simulink model "test_simulation_3_movement"  (R2022a)
settings: Solver=VariableStepAuto  StartTime=0.0  StopTime=1  RelTol=1e-3
libraries: simulink x24, spsMosfetLib x24, spsControlledVoltageSourceLib x4, slpidlib x4, spsPermanentMagnetSynchronousMachineLib x4, spspowerguiLib x1
(part 2 of 2)

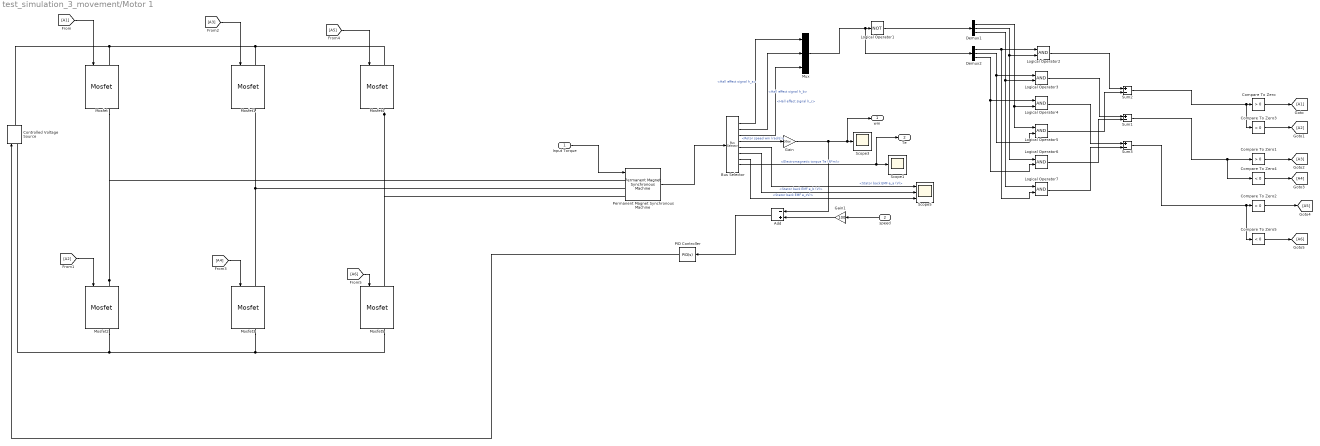
== system test_simulation_3_movement/Motor 1 ==
  Input Torque : Inport
  speed : Inport  Port=2
  Add : Sum  Inputs=-+
  Bus Selector : BusSelector  OutputSignals=Hall effect signal h_a,Hall effect signal h_b,Hall effect signal h_c,Rotor speed wm (rad/s),Stator back EMF e_a (V),Stator back EMF e_b (V),Stator back EMF e_cV),Electromagnetic torque Te (N*m)
  Compare To Zero : simulink/Logic and Bit Operations/Compare To Zero  relop=>  OutDataTypeStr=boolean
  Compare To Zero1 : simulink/Logic and Bit Operations/Compare To Zero  relop=>  OutDataTypeStr=boolean
  Compare To Zero2 : simulink/Logic and Bit Operations/Compare To Zero  relop=>  OutDataTypeStr=boolean
  Compare To Zero3 : simulink/Logic and Bit Operations/Compare To Zero  relop=<  OutDataTypeStr=boolean
  Compare To Zero4 : simulink/Logic and Bit Operations/Compare To Zero  relop=<  OutDataTypeStr=boolean
  Compare To Zero5 : simulink/Logic and Bit Operations/Compare To Zero  relop=<  OutDataTypeStr=boolean
  Controlled Voltage Source : spsControlledVoltageSourceLib/Controlled Voltage Source  Initialize=on  Source_Type=DC  Amplitude=160  Phase=0  Frequency=0  Measurements=None
  Demux1 : Demux  Outputs=3
  Demux2 : Demux  Outputs=3
  Gain : Gain  Gain=30/pi
  Gain1 : Gain  Gain=100
  Logical Operator1 : Logic  Operator=NOT  AllPortsSameDT=off  OutDataTypeStr=boolean
  Logical Operator{2..7} (6 alike) : Logic  AllPortsSameDT=off  OutDataTypeStr=boolean
  Mosfet{,1..5} (6 alike) : spsMosfetLib/Mosfet  Ron=0.1  Lon=0  Rd=0.01  Vfd=0  IC=0  Rs=1e5  Cs=inf  Measurements=on
  Mux : Mux  Inputs=3
  PID Controller : slpidlib/PID Controller  Controller=PID  Form=Parallel  TimeDomain=Continuous-time  UseExternalTs=off  SampleTime=-1  IntegratorMethod=Forward Euler  FilterMethod=Forward Euler  ControllerParametersSource=internal  P=0.01035  I=12.777  UseKiTs=off  D=12.564  N=0  UseFilter=on  TunerSelectOption=Transfer Function Based (PID Tuner App)  InitialConditionSource=internal  InitialConditionForIntegrator=0  InitialConditionForFilter=0  DifferentiatorICPrevScaledInput=0  ExternalReset=none  TrackingMode=off  Kt=1  LimitOutput=off  SatLimitsSource=internal  UpperSaturationLimit=inf  LowerSaturationLimit=-inf  LinearizeAsGain=on  AntiWindupMode=none  Kb=1  POutMin=[]  POutMax=[]  IOutMin=[]  IOutMax=[]  DOutMin=[]  DOutMax=[]  NOutMin=[]  NOutMax=[]  SumOutMin=[]  SumOutMax=[]  SaturationOutMin=[]  SaturationOutMax=[]  PParamMin=[]  PParamMax=[]  IParamMin=[]  IParamMax=[]  DParamMin=[]  DParamMax=[]  NParamMin=[]  NParamMax=[]  KbParamMin=[]  KbParamMax=[]  KtParamMin=[]  KtParamMax=[]  KbOutMin=[]  KbOutMax=[]  KtOutMin=[]  KtOutMax=[]  IntegratorOutMin=[]  IntegratorOutMax=[]  FilterOutMin=[]  FilterOutMax=[]  SumI1OutMin=[]  SumI1OutMax=[]  SumI2OutMin=[]  SumI2OutMax=[]  SumI3OutMin=[]  SumI3OutMax=[]  SumI4OutMin=[]  SumI4OutMax=[]  SumDOutMin=[]  SumDOutMax=[]  DifferentiatorOutMin=[]  DifferentiatorOutMax=[]  FilterDiffOutCoefMin=[]  FilterDiffOutCoefMax=[]  ReciprocalOutMin=[]  ReciprocalOutMax=[]  SumDenOutMin=[]  SumDenOutMax=[]  SumNumOutMin=[]  SumNumOutMax=[]  DivideOutMin=[]  DivideOutMax=[]  UdiffTsProdOutMin=[]  UdiffTsProdOutMax=[]  NTsProdOutMin=[]  NTsProdOutMax=[]  UintegralTsProdOutMin=[]  UintegralTsProdOutMax=[]  UngainTsProdOutMin=[]  UngainTsProdOutMax=[]  IntegratorContinuousStateAttributes=''  IntegratorStateMustResolveToSignalObject=off  IntegratorRTWStateStorageClass=Auto  FilterContinuousStateAttributes=''  FilterStateMustResolveToSignalObject=off  FilterRTWStateStorageClass=Auto  ParallelPVariant=InternalParameters  IdealPVariant=Disabled  IVariant=InternalParameters  DVariant=InternalParameters  IntegratorVariant=Continuous  SatVariant=Disabled  AWVariant=Passthrough  PCopyVariant=Disabled  TRVariant=Disabled  FdbkBlocksVariant=Forward  IdealPFdbkVariant=Disabled  SatFdbkVariant=Disabled  DerivativeFilterVariant=ContFilter  NVariant=InternalParameters  NCopyVariant=Disabled  FilterICVariant=InternalICsFilter  IntegratorICVariant=InternalICs  ExternalResetVariant=Disabled  TRSumVariant=Passthrough  SumFdbkVariant=Disabled  SumVariant=Sum_PID  TsampFilterVariant=InternalTs  TsampNgainVariant=Passthrough  TsampIntegralVariant=Passthrough  ExternalSaturationOutDataTypeStr=Inherit: Same as second input  aMode=0
  Permanent Magnet Synchronous Machine : spsPermanentMagnetSynchronousMachineLib/Permanent Magnet Synchronous Machine  NbPhases=3  FluxDistribution=Trapezoidal  RotorType=Round  MechanicalLoad=Torque Tm  PresetModel=No  ShowDetailedParameters=on  MeasurementBus=off  Resistance=0.7  Inductance=2.7e-3  dqInductances=[8.5e-3,8.5e-3]  La=0.000395  MachineConstant=Flux linkage established by magnets (V.s)  Flux=0.1194  VoltageCst=100.0283  TorqueCst=0.9552  Flat=120  Mechanical=[0.0027 0.0004924 4 0]  PolePairs=4  InitialConditions=[0,0, 0,0]  InitialConditions5ph=[0 0 0 0 0 0]  RefAngle=90 degrees behind phase A axis (modified Park)  IterativeDiscreteModel=Trapezoidal non iterative  TsBlock=-1  TsPowergui=0
  Scope1 : Scope
  Scope3 : Scope
  Scope5 : Scope  NumInputPorts=3
  Sum1 : Sum  Inputs=+-  OutDataTypeStr=double
  Sum2 : Sum  Inputs=+-  OutDataTypeStr=double
  Sum3 : Sum  Inputs=+-  OutDataTypeStr=double
  wm : Outport
  Te : Outport  Port=2
  wires:
  Sum3/1 -> Compare To Zero5/1, Compare To Zero2/1
  [A5] -> Mosfet4/1
  Compare To Zero5/1 -> [A6]
  Sum1/1 -> Compare To Zero4/1, Compare To Zero1/1
  Logical Operator1/1 -> Demux1/1
  Compare To Zero1/1 -> [A3]
  Compare To Zero4/1 -> [A4]
  Logical Operator6/1 -> Sum1/2
  Compare To Zero3/1 -> [A2]
  Demux1/1 -> Logical Operator4/2, Logical Operator5/1
  Demux2/1 -> Logical Operator7/2, Logical Operator2/1
  Gain/1 -> Add/1, wm/1, Scope3/1
  Bus Selector/2 -> Mux/2  "<Hall effect signal h_b>"
  Sum2/1 -> Compare To Zero3/1, Compare To Zero/1
  [A4] -> Mosfet3/1
  Bus Selector/3 -> Mux/3  "<Hall effect signal h_c>"
  [A3] -> Mosfet1/1
  PID Controller/1 -> Controlled Voltage Source/1
  [A1] -> Mosfet/1
  Logical Operator7/1 -> Sum3/2
  Mux/1 -> Demux2/1, Logical Operator1/1
  Bus Selector/8 -> Te/1, Scope1/1  "<Electromagnetic torque Te (N*m)>"
  Bus Selector/4 -> Gain/1  "<Rotor speed wm (rad/s)>"
  [A6] -> Mosfet5/1
  Compare To Zero/1 -> [A1]
  Demux1/2 -> Logical Operator6/1, Logical Operator2/2
  Compare To Zero2/1 -> [A5]
  Logical Operator5/1 -> Sum2/2
  Logical Operator2/1 -> Sum2/1
  Bus Selector/1 -> Mux/1  "<Hall effect signal h_a>"
  Permanent Magnet Synchronous Machine/1 -> Bus Selector/1
  Add/1 -> PID Controller/1
  Bus Selector/7 -> Scope5/3  "<Stator back EMF e_cV)>"
  Logical Operator4/1 -> Sum3/1
  Logical Operator3/1 -> Sum1/1
  Demux1/3 -> Logical Operator7/1, Logical Operator3/2
  Demux2/3 -> Logical Operator4/1, Logical Operator6/2
  [A2] -> Mosfet2/1
  Demux2/2 -> Logical Operator3/1, Logical Operator5/2
  Bus Selector/5 -> Scope5/1  "<Stator back EMF e_a (V)>"
  Bus Selector/6 -> Scope5/2  "<Stator back EMF e_b (V)>"
  Input Torque/1 -> Permanent Magnet Synchronous Machine/1
  speed/1 -> Gain1/1
  Gain1/1 -> Add/2
  connections:
  Mosfet3/RConn1 -- Mosfet5/RConn1 -- Controlled Voltage Source/LConn1 -- Mosfet2/RConn1
  Mosfet1/LConn1 -- Controlled Voltage Source/RConn1 -- Mosfet/LConn1 -- Mosfet4/LConn1
  Mosfet4/RConn1 -- Mosfet5/LConn1 -- Permanent Magnet Synchronous Machine/LConn3
  Mosfet2/LConn1 -- Mosfet/RConn1 -- Permanent Magnet Synchronous Machine/LConn1
  Mosfet3/LConn1 -- Mosfet1/RConn1 -- Permanent Magnet Synchronous Machine/LConn2

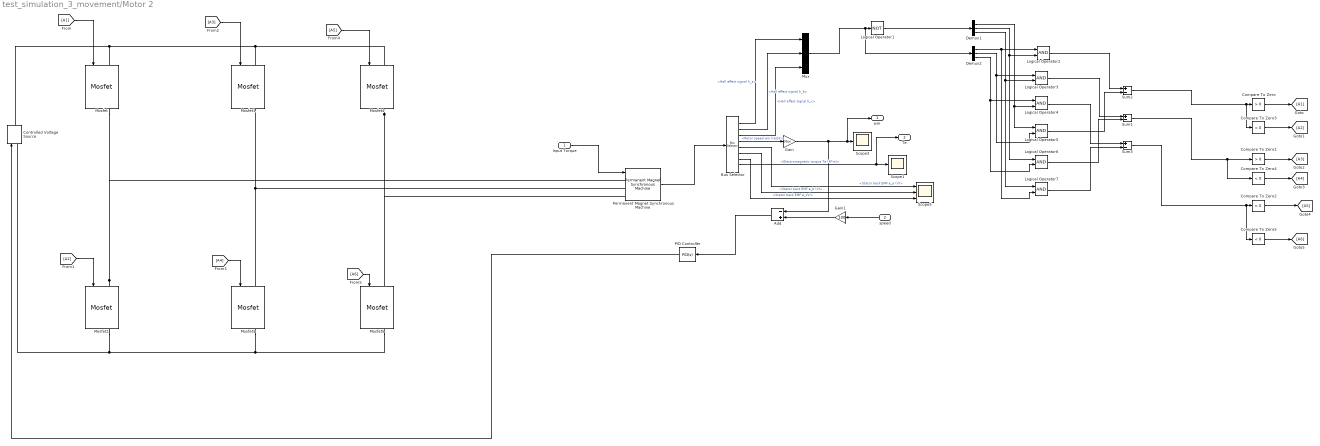
== system test_simulation_3_movement/Motor 2 ==
  Input Torque : Inport
  speed : Inport  Port=2
  Add : Sum  Inputs=-+
  Bus Selector : BusSelector  OutputSignals=Hall effect signal h_a,Hall effect signal h_b,Hall effect signal h_c,Rotor speed wm (rad/s),Stator back EMF e_a (V),Stator back EMF e_b (V),Stator back EMF e_cV),Electromagnetic torque Te (N*m)
  Compare To Zero : simulink/Logic and Bit Operations/Compare To Zero  relop=>  OutDataTypeStr=boolean
  Compare To Zero1 : simulink/Logic and Bit Operations/Compare To Zero  relop=>  OutDataTypeStr=boolean
  Compare To Zero2 : simulink/Logic and Bit Operations/Compare To Zero  relop=>  OutDataTypeStr=boolean
  Compare To Zero3 : simulink/Logic and Bit Operations/Compare To Zero  relop=<  OutDataTypeStr=boolean
  Compare To Zero4 : simulink/Logic and Bit Operations/Compare To Zero  relop=<  OutDataTypeStr=boolean
  Compare To Zero5 : simulink/Logic and Bit Operations/Compare To Zero  relop=<  OutDataTypeStr=boolean
  Controlled Voltage Source : spsControlledVoltageSourceLib/Controlled Voltage Source  Initialize=on  Source_Type=DC  Amplitude=160  Phase=0  Frequency=0  Measurements=None
  Demux1 : Demux  Outputs=3
  Demux2 : Demux  Outputs=3
  Gain : Gain  Gain=30/pi
  Gain1 : Gain  Gain=100
  Logical Operator1 : Logic  Operator=NOT  AllPortsSameDT=off  OutDataTypeStr=boolean
  Logical Operator{2..7} (6 alike) : Logic  AllPortsSameDT=off  OutDataTypeStr=boolean
  Mosfet{,1..5} (6 alike) : spsMosfetLib/Mosfet  Ron=0.1  Lon=0  Rd=0.01  Vfd=0  IC=0  Rs=1e5  Cs=inf  Measurements=on
  Mux : Mux  Inputs=3
  PID Controller : slpidlib/PID Controller  Controller=PID  Form=Parallel  TimeDomain=Continuous-time  UseExternalTs=off  SampleTime=-1  IntegratorMethod=Forward Euler  FilterMethod=Forward Euler  ControllerParametersSource=internal  P=0.01035  I=12.777  UseKiTs=off  D=12.564  N=0  UseFilter=on  TunerSelectOption=Transfer Function Based (PID Tuner App)  InitialConditionSource=internal  InitialConditionForIntegrator=0  InitialConditionForFilter=0  DifferentiatorICPrevScaledInput=0  ExternalReset=none  TrackingMode=off  Kt=1  LimitOutput=off  SatLimitsSource=internal  UpperSaturationLimit=inf  LowerSaturationLimit=-inf  LinearizeAsGain=on  AntiWindupMode=none  Kb=1  POutMin=[]  POutMax=[]  IOutMin=[]  IOutMax=[]  DOutMin=[]  DOutMax=[]  NOutMin=[]  NOutMax=[]  SumOutMin=[]  SumOutMax=[]  SaturationOutMin=[]  SaturationOutMax=[]  PParamMin=[]  PParamMax=[]  IParamMin=[]  IParamMax=[]  DParamMin=[]  DParamMax=[]  NParamMin=[]  NParamMax=[]  KbParamMin=[]  KbParamMax=[]  KtParamMin=[]  KtParamMax=[]  KbOutMin=[]  KbOutMax=[]  KtOutMin=[]  KtOutMax=[]  IntegratorOutMin=[]  IntegratorOutMax=[]  FilterOutMin=[]  FilterOutMax=[]  SumI1OutMin=[]  SumI1OutMax=[]  SumI2OutMin=[]  SumI2OutMax=[]  SumI3OutMin=[]  SumI3OutMax=[]  SumI4OutMin=[]  SumI4OutMax=[]  SumDOutMin=[]  SumDOutMax=[]  DifferentiatorOutMin=[]  DifferentiatorOutMax=[]  FilterDiffOutCoefMin=[]  FilterDiffOutCoefMax=[]  ReciprocalOutMin=[]  ReciprocalOutMax=[]  SumDenOutMin=[]  SumDenOutMax=[]  SumNumOutMin=[]  SumNumOutMax=[]  DivideOutMin=[]  DivideOutMax=[]  UdiffTsProdOutMin=[]  UdiffTsProdOutMax=[]  NTsProdOutMin=[]  NTsProdOutMax=[]  UintegralTsProdOutMin=[]  UintegralTsProdOutMax=[]  UngainTsProdOutMin=[]  UngainTsProdOutMax=[]  IntegratorContinuousStateAttributes=''  IntegratorStateMustResolveToSignalObject=off  IntegratorRTWStateStorageClass=Auto  FilterContinuousStateAttributes=''  FilterStateMustResolveToSignalObject=off  FilterRTWStateStorageClass=Auto  ParallelPVariant=InternalParameters  IdealPVariant=Disabled  IVariant=InternalParameters  DVariant=InternalParameters  IntegratorVariant=Continuous  SatVariant=Disabled  AWVariant=Passthrough  PCopyVariant=Disabled  TRVariant=Disabled  FdbkBlocksVariant=Forward  IdealPFdbkVariant=Disabled  SatFdbkVariant=Disabled  DerivativeFilterVariant=ContFilter  NVariant=InternalParameters  NCopyVariant=Disabled  FilterICVariant=InternalICsFilter  IntegratorICVariant=InternalICs  ExternalResetVariant=Disabled  TRSumVariant=Passthrough  SumFdbkVariant=Disabled  SumVariant=Sum_PID  TsampFilterVariant=InternalTs  TsampNgainVariant=Passthrough  TsampIntegralVariant=Passthrough  ExternalSaturationOutDataTypeStr=Inherit: Same as second input  aMode=0
  Permanent Magnet Synchronous Machine : spsPermanentMagnetSynchronousMachineLib/Permanent Magnet Synchronous Machine  NbPhases=3  FluxDistribution=Trapezoidal  RotorType=Round  MechanicalLoad=Torque Tm  PresetModel=No  ShowDetailedParameters=on  MeasurementBus=off  Resistance=0.7  Inductance=2.7e-3  dqInductances=[8.5e-3,8.5e-3]  La=0.000395  MachineConstant=Flux linkage established by magnets (V.s)  Flux=0.1194  VoltageCst=100.0283  TorqueCst=0.9552  Flat=120  Mechanical=[0.0027 0.0004924 4 0]  PolePairs=4  InitialConditions=[0,0, 0,0]  InitialConditions5ph=[0 0 0 0 0 0]  RefAngle=90 degrees behind phase A axis (modified Park)  IterativeDiscreteModel=Trapezoidal non iterative  TsBlock=-1  TsPowergui=0
  Scope1 : Scope
  Scope3 : Scope
  Scope5 : Scope  NumInputPorts=3
  Sum1 : Sum  Inputs=+-  OutDataTypeStr=double
  Sum2 : Sum  Inputs=+-  OutDataTypeStr=double
  Sum3 : Sum  Inputs=+-  OutDataTypeStr=double
  wm : Outport
  Te : Outport  Port=2
  wires:
  Sum3/1 -> Compare To Zero5/1, Compare To Zero2/1
  [A5] -> Mosfet4/1
  Compare To Zero5/1 -> [A6]
  Sum1/1 -> Compare To Zero4/1, Compare To Zero1/1
  Logical Operator1/1 -> Demux1/1
  Compare To Zero1/1 -> [A3]
  Compare To Zero4/1 -> [A4]
  Logical Operator6/1 -> Sum1/2
  Compare To Zero3/1 -> [A2]
  Demux1/1 -> Logical Operator4/2, Logical Operator5/1
  Demux2/1 -> Logical Operator7/2, Logical Operator2/1
  Gain/1 -> Add/1, wm/1, Scope3/1
  Bus Selector/2 -> Mux/2  "<Hall effect signal h_b>"
  Sum2/1 -> Compare To Zero3/1, Compare To Zero/1
  [A4] -> Mosfet3/1
  Bus Selector/3 -> Mux/3  "<Hall effect signal h_c>"
  [A3] -> Mosfet1/1
  PID Controller/1 -> Controlled Voltage Source/1
  [A1] -> Mosfet/1
  Logical Operator7/1 -> Sum3/2
  Mux/1 -> Demux2/1, Logical Operator1/1
  Bus Selector/8 -> Te/1, Scope1/1  "<Electromagnetic torque Te (N*m)>"
  Bus Selector/4 -> Gain/1  "<Rotor speed wm (rad/s)>"
  [A6] -> Mosfet5/1
  Compare To Zero/1 -> [A1]
  Demux1/2 -> Logical Operator6/1, Logical Operator2/2
  Compare To Zero2/1 -> [A5]
  Logical Operator5/1 -> Sum2/2
  Logical Operator2/1 -> Sum2/1
  Bus Selector/1 -> Mux/1  "<Hall effect signal h_a>"
  Permanent Magnet Synchronous Machine/1 -> Bus Selector/1
  Add/1 -> PID Controller/1
  Bus Selector/7 -> Scope5/3  "<Stator back EMF e_cV)>"
  Logical Operator4/1 -> Sum3/1
  Logical Operator3/1 -> Sum1/1
  Demux1/3 -> Logical Operator7/1, Logical Operator3/2
  Demux2/3 -> Logical Operator4/1, Logical Operator6/2
  [A2] -> Mosfet2/1
  Demux2/2 -> Logical Operator3/1, Logical Operator5/2
  Bus Selector/5 -> Scope5/1  "<Stator back EMF e_a (V)>"
  Bus Selector/6 -> Scope5/2  "<Stator back EMF e_b (V)>"
  Input Torque/1 -> Permanent Magnet Synchronous Machine/1
  speed/1 -> Gain1/1
  Gain1/1 -> Add/2
  connections:
  Mosfet3/RConn1 -- Mosfet5/RConn1 -- Controlled Voltage Source/LConn1 -- Mosfet2/RConn1
  Mosfet1/LConn1 -- Controlled Voltage Source/RConn1 -- Mosfet/LConn1 -- Mosfet4/LConn1
  Mosfet4/RConn1 -- Mosfet5/LConn1 -- Permanent Magnet Synchronous Machine/LConn3
  Mosfet2/LConn1 -- Mosfet/RConn1 -- Permanent Magnet Synchronous Machine/LConn1
  Mosfet3/LConn1 -- Mosfet1/RConn1 -- Permanent Magnet Synchronous Machine/LConn2

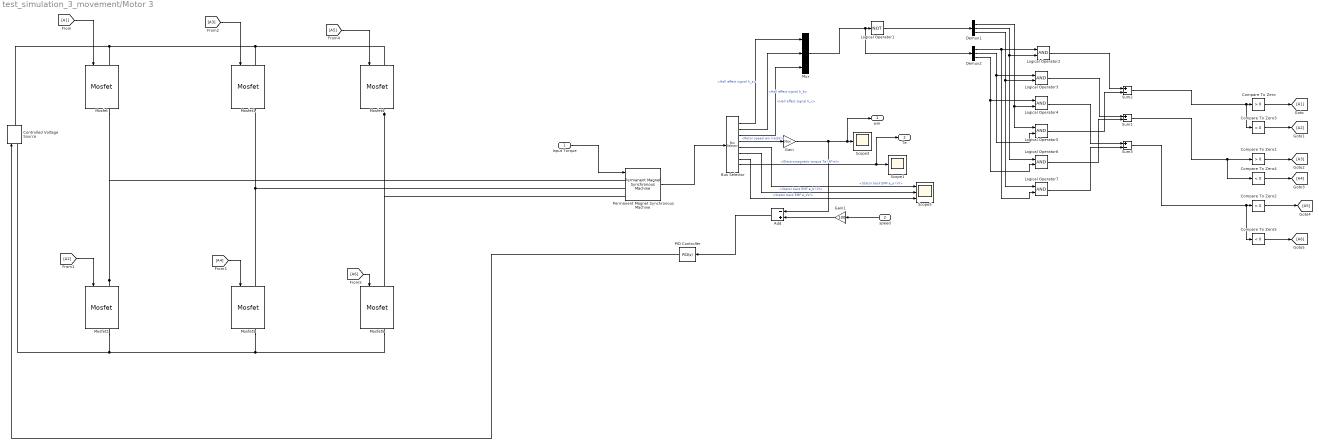
== system test_simulation_3_movement/Motor 3 ==
  Input Torque : Inport
  speed : Inport  Port=2
  Add : Sum  Inputs=-+
  Bus Selector : BusSelector  OutputSignals=Hall effect signal h_a,Hall effect signal h_b,Hall effect signal h_c,Rotor speed wm (rad/s),Stator back EMF e_a (V),Stator back EMF e_b (V),Stator back EMF e_cV),Electromagnetic torque Te (N*m)
  Compare To Zero : simulink/Logic and Bit Operations/Compare To Zero  relop=>  OutDataTypeStr=boolean
  Compare To Zero1 : simulink/Logic and Bit Operations/Compare To Zero  relop=>  OutDataTypeStr=boolean
  Compare To Zero2 : simulink/Logic and Bit Operations/Compare To Zero  relop=>  OutDataTypeStr=boolean
  Compare To Zero3 : simulink/Logic and Bit Operations/Compare To Zero  relop=<  OutDataTypeStr=boolean
  Compare To Zero4 : simulink/Logic and Bit Operations/Compare To Zero  relop=<  OutDataTypeStr=boolean
  Compare To Zero5 : simulink/Logic and Bit Operations/Compare To Zero  relop=<  OutDataTypeStr=boolean
  Controlled Voltage Source : spsControlledVoltageSourceLib/Controlled Voltage Source  Initialize=on  Source_Type=DC  Amplitude=160  Phase=0  Frequency=0  Measurements=None
  Demux1 : Demux  Outputs=3
  Demux2 : Demux  Outputs=3
  Gain : Gain  Gain=30/pi
  Gain1 : Gain  Gain=100
  Logical Operator1 : Logic  Operator=NOT  AllPortsSameDT=off  OutDataTypeStr=boolean
  Logical Operator{2..7} (6 alike) : Logic  AllPortsSameDT=off  OutDataTypeStr=boolean
  Mosfet{,1..5} (6 alike) : spsMosfetLib/Mosfet  Ron=0.1  Lon=0  Rd=0.01  Vfd=0  IC=0  Rs=1e5  Cs=inf  Measurements=on
  Mux : Mux  Inputs=3
  PID Controller : slpidlib/PID Controller  Controller=PID  Form=Parallel  TimeDomain=Continuous-time  UseExternalTs=off  SampleTime=-1  IntegratorMethod=Forward Euler  FilterMethod=Forward Euler  ControllerParametersSource=internal  P=0.01035  I=12.777  UseKiTs=off  D=12.564  N=0  UseFilter=on  TunerSelectOption=Transfer Function Based (PID Tuner App)  InitialConditionSource=internal  InitialConditionForIntegrator=0  InitialConditionForFilter=0  DifferentiatorICPrevScaledInput=0  ExternalReset=none  TrackingMode=off  Kt=1  LimitOutput=off  SatLimitsSource=internal  UpperSaturationLimit=inf  LowerSaturationLimit=-inf  LinearizeAsGain=on  AntiWindupMode=none  Kb=1  POutMin=[]  POutMax=[]  IOutMin=[]  IOutMax=[]  DOutMin=[]  DOutMax=[]  NOutMin=[]  NOutMax=[]  SumOutMin=[]  SumOutMax=[]  SaturationOutMin=[]  SaturationOutMax=[]  PParamMin=[]  PParamMax=[]  IParamMin=[]  IParamMax=[]  DParamMin=[]  DParamMax=[]  NParamMin=[]  NParamMax=[]  KbParamMin=[]  KbParamMax=[]  KtParamMin=[]  KtParamMax=[]  KbOutMin=[]  KbOutMax=[]  KtOutMin=[]  KtOutMax=[]  IntegratorOutMin=[]  IntegratorOutMax=[]  FilterOutMin=[]  FilterOutMax=[]  SumI1OutMin=[]  SumI1OutMax=[]  SumI2OutMin=[]  SumI2OutMax=[]  SumI3OutMin=[]  SumI3OutMax=[]  SumI4OutMin=[]  SumI4OutMax=[]  SumDOutMin=[]  SumDOutMax=[]  DifferentiatorOutMin=[]  DifferentiatorOutMax=[]  FilterDiffOutCoefMin=[]  FilterDiffOutCoefMax=[]  ReciprocalOutMin=[]  ReciprocalOutMax=[]  SumDenOutMin=[]  SumDenOutMax=[]  SumNumOutMin=[]  SumNumOutMax=[]  DivideOutMin=[]  DivideOutMax=[]  UdiffTsProdOutMin=[]  UdiffTsProdOutMax=[]  NTsProdOutMin=[]  NTsProdOutMax=[]  UintegralTsProdOutMin=[]  UintegralTsProdOutMax=[]  UngainTsProdOutMin=[]  UngainTsProdOutMax=[]  IntegratorContinuousStateAttributes=''  IntegratorStateMustResolveToSignalObject=off  IntegratorRTWStateStorageClass=Auto  FilterContinuousStateAttributes=''  FilterStateMustResolveToSignalObject=off  FilterRTWStateStorageClass=Auto  ParallelPVariant=InternalParameters  IdealPVariant=Disabled  IVariant=InternalParameters  DVariant=InternalParameters  IntegratorVariant=Continuous  SatVariant=Disabled  AWVariant=Passthrough  PCopyVariant=Disabled  TRVariant=Disabled  FdbkBlocksVariant=Forward  IdealPFdbkVariant=Disabled  SatFdbkVariant=Disabled  DerivativeFilterVariant=ContFilter  NVariant=InternalParameters  NCopyVariant=Disabled  FilterICVariant=InternalICsFilter  IntegratorICVariant=InternalICs  ExternalResetVariant=Disabled  TRSumVariant=Passthrough  SumFdbkVariant=Disabled  SumVariant=Sum_PID  TsampFilterVariant=InternalTs  TsampNgainVariant=Passthrough  TsampIntegralVariant=Passthrough  ExternalSaturationOutDataTypeStr=Inherit: Same as second input  aMode=0
  Permanent Magnet Synchronous Machine : spsPermanentMagnetSynchronousMachineLib/Permanent Magnet Synchronous Machine  NbPhases=3  FluxDistribution=Trapezoidal  RotorType=Round  MechanicalLoad=Torque Tm  PresetModel=No  ShowDetailedParameters=on  MeasurementBus=off  Resistance=0.7  Inductance=2.7e-3  dqInductances=[8.5e-3,8.5e-3]  La=0.000395  MachineConstant=Flux linkage established by magnets (V.s)  Flux=0.1194  VoltageCst=100.0283  TorqueCst=0.9552  Flat=120  Mechanical=[0.0027 0.0004924 4 0]  PolePairs=4  InitialConditions=[0,0, 0,0]  InitialConditions5ph=[0 0 0 0 0 0]  RefAngle=90 degrees behind phase A axis (modified Park)  IterativeDiscreteModel=Trapezoidal non iterative  TsBlock=-1  TsPowergui=0
  Scope1 : Scope
  Scope3 : Scope
  Scope5 : Scope  NumInputPorts=3
  Sum1 : Sum  Inputs=+-  OutDataTypeStr=double
  Sum2 : Sum  Inputs=+-  OutDataTypeStr=double
  Sum3 : Sum  Inputs=+-  OutDataTypeStr=double
  wm : Outport
  Te : Outport  Port=2
  wires:
  Sum3/1 -> Compare To Zero5/1, Compare To Zero2/1
  [A5] -> Mosfet4/1
  Compare To Zero5/1 -> [A6]
  Sum1/1 -> Compare To Zero4/1, Compare To Zero1/1
  Logical Operator1/1 -> Demux1/1
  Compare To Zero1/1 -> [A3]
  Compare To Zero4/1 -> [A4]
  Logical Operator6/1 -> Sum1/2
  Compare To Zero3/1 -> [A2]
  Demux1/1 -> Logical Operator4/2, Logical Operator5/1
  Demux2/1 -> Logical Operator7/2, Logical Operator2/1
  Gain/1 -> Add/1, wm/1, Scope3/1
  Bus Selector/2 -> Mux/2  "<Hall effect signal h_b>"
  Sum2/1 -> Compare To Zero3/1, Compare To Zero/1
  [A4] -> Mosfet3/1
  Bus Selector/3 -> Mux/3  "<Hall effect signal h_c>"
  [A3] -> Mosfet1/1
  PID Controller/1 -> Controlled Voltage Source/1
  [A1] -> Mosfet/1
  Logical Operator7/1 -> Sum3/2
  Mux/1 -> Demux2/1, Logical Operator1/1
  Bus Selector/8 -> Te/1, Scope1/1  "<Electromagnetic torque Te (N*m)>"
  Bus Selector/4 -> Gain/1  "<Rotor speed wm (rad/s)>"
  [A6] -> Mosfet5/1
  Compare To Zero/1 -> [A1]
  Demux1/2 -> Logical Operator6/1, Logical Operator2/2
  Compare To Zero2/1 -> [A5]
  Logical Operator5/1 -> Sum2/2
  Logical Operator2/1 -> Sum2/1
  Bus Selector/1 -> Mux/1  "<Hall effect signal h_a>"
  Permanent Magnet Synchronous Machine/1 -> Bus Selector/1
  Add/1 -> PID Controller/1
  Bus Selector/7 -> Scope5/3  "<Stator back EMF e_cV)>"
  Logical Operator4/1 -> Sum3/1
  Logical Operator3/1 -> Sum1/1
  Demux1/3 -> Logical Operator7/1, Logical Operator3/2
  Demux2/3 -> Logical Operator4/1, Logical Operator6/2
  [A2] -> Mosfet2/1
  Demux2/2 -> Logical Operator3/1, Logical Operator5/2
  Bus Selector/5 -> Scope5/1  "<Stator back EMF e_a (V)>"
  Bus Selector/6 -> Scope5/2  "<Stator back EMF e_b (V)>"
  Input Torque/1 -> Permanent Magnet Synchronous Machine/1
  speed/1 -> Gain1/1
  Gain1/1 -> Add/2
  connections:
  Mosfet3/RConn1 -- Mosfet5/RConn1 -- Controlled Voltage Source/LConn1 -- Mosfet2/RConn1
  Mosfet1/LConn1 -- Controlled Voltage Source/RConn1 -- Mosfet/LConn1 -- Mosfet4/LConn1
  Mosfet4/RConn1 -- Mosfet5/LConn1 -- Permanent Magnet Synchronous Machine/LConn3
  Mosfet2/LConn1 -- Mosfet/RConn1 -- Permanent Magnet Synchronous Machine/LConn1
  Mosfet3/LConn1 -- Mosfet1/RConn1 -- Permanent Magnet Synchronous Machine/LConn2

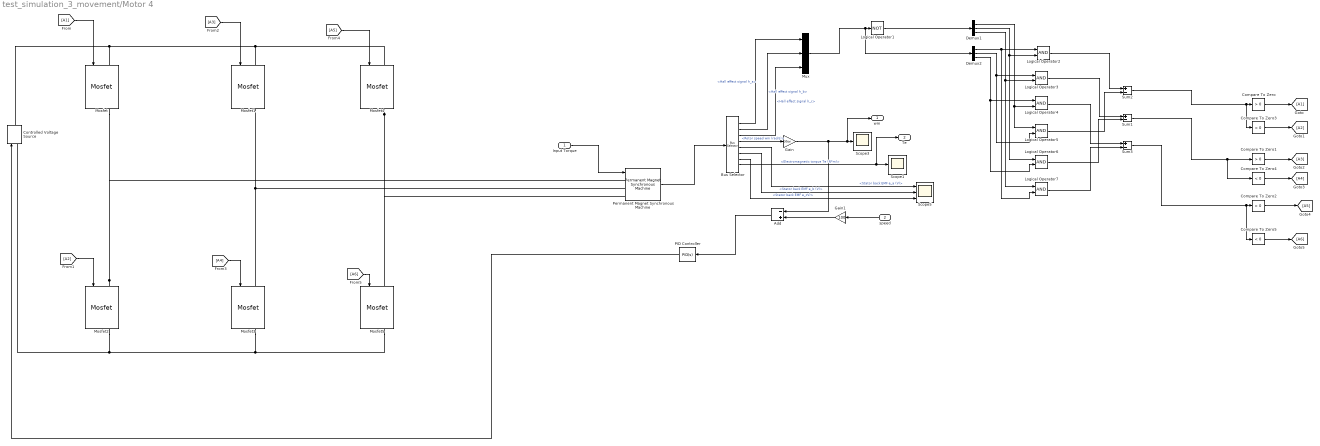
== system test_simulation_3_movement/Motor 4 ==
  Input Torque : Inport
  speed : Inport  Port=2
  Add : Sum  Inputs=-+
  Bus Selector : BusSelector  OutputSignals=Hall effect signal h_a,Hall effect signal h_b,Hall effect signal h_c,Rotor speed wm (rad/s),Stator back EMF e_a (V),Stator back EMF e_b (V),Stator back EMF e_cV),Electromagnetic torque Te (N*m)
  Compare To Zero : simulink/Logic and Bit Operations/Compare To Zero  relop=>  OutDataTypeStr=boolean
  Compare To Zero1 : simulink/Logic and Bit Operations/Compare To Zero  relop=>  OutDataTypeStr=boolean
  Compare To Zero2 : simulink/Logic and Bit Operations/Compare To Zero  relop=>  OutDataTypeStr=boolean
  Compare To Zero3 : simulink/Logic and Bit Operations/Compare To Zero  relop=<  OutDataTypeStr=boolean
  Compare To Zero4 : simulink/Logic and Bit Operations/Compare To Zero  relop=<  OutDataTypeStr=boolean
  Compare To Zero5 : simulink/Logic and Bit Operations/Compare To Zero  relop=<  OutDataTypeStr=boolean
  Controlled Voltage Source : spsControlledVoltageSourceLib/Controlled Voltage Source  Initialize=on  Source_Type=DC  Amplitude=160  Phase=0  Frequency=0  Measurements=None
  Demux1 : Demux  Outputs=3
  Demux2 : Demux  Outputs=3
  Gain : Gain  Gain=30/pi
  Gain1 : Gain  Gain=100
  Logical Operator1 : Logic  Operator=NOT  AllPortsSameDT=off  OutDataTypeStr=boolean
  Logical Operator{2..7} (6 alike) : Logic  AllPortsSameDT=off  OutDataTypeStr=boolean
  Mosfet{,1..5} (6 alike) : spsMosfetLib/Mosfet  Ron=0.1  Lon=0  Rd=0.01  Vfd=0  IC=0  Rs=1e5  Cs=inf  Measurements=on
  Mux : Mux  Inputs=3
  PID Controller : slpidlib/PID Controller  Controller=PID  Form=Parallel  TimeDomain=Continuous-time  UseExternalTs=off  SampleTime=-1  IntegratorMethod=Forward Euler  FilterMethod=Forward Euler  ControllerParametersSource=internal  P=0.01035  I=12.777  UseKiTs=off  D=12.564  N=0  UseFilter=on  TunerSelectOption=Transfer Function Based (PID Tuner App)  InitialConditionSource=internal  InitialConditionForIntegrator=0  InitialConditionForFilter=0  DifferentiatorICPrevScaledInput=0  ExternalReset=none  TrackingMode=off  Kt=1  LimitOutput=off  SatLimitsSource=internal  UpperSaturationLimit=inf  LowerSaturationLimit=-inf  LinearizeAsGain=on  AntiWindupMode=none  Kb=1  POutMin=[]  POutMax=[]  IOutMin=[]  IOutMax=[]  DOutMin=[]  DOutMax=[]  NOutMin=[]  NOutMax=[]  SumOutMin=[]  SumOutMax=[]  SaturationOutMin=[]  SaturationOutMax=[]  PParamMin=[]  PParamMax=[]  IParamMin=[]  IParamMax=[]  DParamMin=[]  DParamMax=[]  NParamMin=[]  NParamMax=[]  KbParamMin=[]  KbParamMax=[]  KtParamMin=[]  KtParamMax=[]  KbOutMin=[]  KbOutMax=[]  KtOutMin=[]  KtOutMax=[]  IntegratorOutMin=[]  IntegratorOutMax=[]  FilterOutMin=[]  FilterOutMax=[]  SumI1OutMin=[]  SumI1OutMax=[]  SumI2OutMin=[]  SumI2OutMax=[]  SumI3OutMin=[]  SumI3OutMax=[]  SumI4OutMin=[]  SumI4OutMax=[]  SumDOutMin=[]  SumDOutMax=[]  DifferentiatorOutMin=[]  DifferentiatorOutMax=[]  FilterDiffOutCoefMin=[]  FilterDiffOutCoefMax=[]  ReciprocalOutMin=[]  ReciprocalOutMax=[]  SumDenOutMin=[]  SumDenOutMax=[]  SumNumOutMin=[]  SumNumOutMax=[]  DivideOutMin=[]  DivideOutMax=[]  UdiffTsProdOutMin=[]  UdiffTsProdOutMax=[]  NTsProdOutMin=[]  NTsProdOutMax=[]  UintegralTsProdOutMin=[]  UintegralTsProdOutMax=[]  UngainTsProdOutMin=[]  UngainTsProdOutMax=[]  IntegratorContinuousStateAttributes=''  IntegratorStateMustResolveToSignalObject=off  IntegratorRTWStateStorageClass=Auto  FilterContinuousStateAttributes=''  FilterStateMustResolveToSignalObject=off  FilterRTWStateStorageClass=Auto  ParallelPVariant=InternalParameters  IdealPVariant=Disabled  IVariant=InternalParameters  DVariant=InternalParameters  IntegratorVariant=Continuous  SatVariant=Disabled  AWVariant=Passthrough  PCopyVariant=Disabled  TRVariant=Disabled  FdbkBlocksVariant=Forward  IdealPFdbkVariant=Disabled  SatFdbkVariant=Disabled  DerivativeFilterVariant=ContFilter  NVariant=InternalParameters  NCopyVariant=Disabled  FilterICVariant=InternalICsFilter  IntegratorICVariant=InternalICs  ExternalResetVariant=Disabled  TRSumVariant=Passthrough  SumFdbkVariant=Disabled  SumVariant=Sum_PID  TsampFilterVariant=InternalTs  TsampNgainVariant=Passthrough  TsampIntegralVariant=Passthrough  ExternalSaturationOutDataTypeStr=Inherit: Same as second input  aMode=0
  Permanent Magnet Synchronous Machine : spsPermanentMagnetSynchronousMachineLib/Permanent Magnet Synchronous Machine  NbPhases=3  FluxDistribution=Trapezoidal  RotorType=Round  MechanicalLoad=Torque Tm  PresetModel=No  ShowDetailedParameters=on  MeasurementBus=off  Resistance=0.7  Inductance=2.7e-3  dqInductances=[8.5e-3,8.5e-3]  La=0.000395  MachineConstant=Flux linkage established by magnets (V.s)  Flux=0.1194  VoltageCst=100.0283  TorqueCst=0.9552  Flat=120  Mechanical=[0.0027 0.0004924 4 0]  PolePairs=4  InitialConditions=[0,0, 0,0]  InitialConditions5ph=[0 0 0 0 0 0]  RefAngle=90 degrees behind phase A axis (modified Park)  IterativeDiscreteModel=Trapezoidal non iterative  TsBlock=-1  TsPowergui=0
  Scope1 : Scope
  Scope3 : Scope
  Scope5 : Scope  NumInputPorts=3
  Sum1 : Sum  Inputs=+-  OutDataTypeStr=double
  Sum2 : Sum  Inputs=+-  OutDataTypeStr=double
  Sum3 : Sum  Inputs=+-  OutDataTypeStr=double
  wm : Outport
  Te : Outport  Port=2
  wires:
  Sum3/1 -> Compare To Zero5/1, Compare To Zero2/1
  [A5] -> Mosfet4/1
  Compare To Zero5/1 -> [A6]
  Sum1/1 -> Compare To Zero4/1, Compare To Zero1/1
  Logical Operator1/1 -> Demux1/1
  Compare To Zero1/1 -> [A3]
  Compare To Zero4/1 -> [A4]
  Logical Operator6/1 -> Sum1/2
  Compare To Zero3/1 -> [A2]
  Demux1/1 -> Logical Operator4/2, Logical Operator5/1
  Demux2/1 -> Logical Operator7/2, Logical Operator2/1
  Gain/1 -> Add/1, wm/1, Scope3/1
  Bus Selector/2 -> Mux/2  "<Hall effect signal h_b>"
  Sum2/1 -> Compare To Zero3/1, Compare To Zero/1
  [A4] -> Mosfet3/1
  Bus Selector/3 -> Mux/3  "<Hall effect signal h_c>"
  [A3] -> Mosfet1/1
  PID Controller/1 -> Controlled Voltage Source/1
  [A1] -> Mosfet/1
  Logical Operator7/1 -> Sum3/2
  Mux/1 -> Demux2/1, Logical Operator1/1
  Bus Selector/8 -> Te/1, Scope1/1  "<Electromagnetic torque Te (N*m)>"
  Bus Selector/4 -> Gain/1  "<Rotor speed wm (rad/s)>"
  [A6] -> Mosfet5/1
  Compare To Zero/1 -> [A1]
  Demux1/2 -> Logical Operator6/1, Logical Operator2/2
  Compare To Zero2/1 -> [A5]
  Logical Operator5/1 -> Sum2/2
  Logical Operator2/1 -> Sum2/1
  Bus Selector/1 -> Mux/1  "<Hall effect signal h_a>"
  Permanent Magnet Synchronous Machine/1 -> Bus Selector/1
  Add/1 -> PID Controller/1
  Bus Selector/7 -> Scope5/3  "<Stator back EMF e_cV)>"
  Logical Operator4/1 -> Sum3/1
  Logical Operator3/1 -> Sum1/1
  Demux1/3 -> Logical Operator7/1, Logical Operator3/2
  Demux2/3 -> Logical Operator4/1, Logical Operator6/2
  [A2] -> Mosfet2/1
  Demux2/2 -> Logical Operator3/1, Logical Operator5/2
  Bus Selector/5 -> Scope5/1  "<Stator back EMF e_a (V)>"
  Bus Selector/6 -> Scope5/2  "<Stator back EMF e_b (V)>"
  Input Torque/1 -> Permanent Magnet Synchronous Machine/1
  speed/1 -> Gain1/1
  Gain1/1 -> Add/2
  connections:
  Mosfet3/RConn1 -- Mosfet5/RConn1 -- Controlled Voltage Source/LConn1 -- Mosfet2/RConn1
  Mosfet1/LConn1 -- Controlled Voltage Source/RConn1 -- Mosfet/LConn1 -- Mosfet4/LConn1
  Mosfet4/RConn1 -- Mosfet5/LConn1 -- Permanent Magnet Synchronous Machine/LConn3
  Mosfet2/LConn1 -- Mosfet/RConn1 -- Permanent Magnet Synchronous Machine/LConn1
  Mosfet3/LConn1 -- Mosfet1/RConn1 -- Permanent Magnet Synchronous Machine/LConn2
